simulink model "scar22"  (R2021a)
settings: Solver=ode23tb  StartTime=0.0  StopTime=.2  RelTol=1e-3
libraries: spsThreePhaseSeriesRLCLoadLib x17, spsThreePhasePISectionLineLib x16, spsThreePhaseTransformerTwoWindingsLib x14, spsThreePhaseVIMeasurementLib x11, simulink x6, exampleMicrogridLibrary x6, spsThreePhaseParallelRLCBranchLib x5, spsThreePhaseDynamicLoadLib x5, spsGroundLib x4, spsAC1AExcitationSystemLib x2, spsDieselMotorModel x2, spsSynchronousMachinepuStandardLib x2
(part 2 of 2)

== system scar22/Variable Load ==
  Load : Inport
  Dynamic Load Control : Subsystem
  Simple Three-Phase Load : spsThreePhaseDynamicLoadLib/Three-Phase Dynamic Load  NominalVoltage=[Vn Fn]  ActiveReactivePowers=[200000 45883.1]  PositiveSequence=[0.999844 -0.0038635]  ExternalControl=on  NpNq=[1.3 2]  TimeConstants="[0  0  0  0]"  MinimumVoltage=0.7  Tfilter=1e-2  LoadFlowParameters=[4,0,0,0,0]
      settings: SourceProductBaseCode=PS
  Terminator : Terminator
  A : PMIOPort  Side=Right
  B : PMIOPort  Port=2  Side=Right
  C : PMIOPort  Port=3  Side=Right
  wires:
  Simple Three-Phase Load/1 -> Terminator/1
  Load/1 -> Dynamic Load Control/1(P0)
  Dynamic Load Control/1(PQ) -> Simple Three-Phase Load/1
  connections:
  Simple Three-Phase Load/LConn1 -- A/RConn1
  Simple Three-Phase Load/LConn3 -- C/RConn1
  Simple Three-Phase Load/LConn2 -- B/RConn1

== system scar22/Diesel Generator1/Generator Measures ==
  m : Inport
  Bus Selector : BusSelector  OutputSignals="dq0 components.Stator voltage  vq (pu),dq0 components.Stator voltage  vd (pu)"  OutputAsBus=on
  Bus Selector1 : BusSelector  OutputSignals="Mechanical.Rotor speed  wm  (pu),dq0 components.Field current  ifd (pu)"
  Fcn1 : Fcn  Expr=sqrt(u(1)^2 + u(2)^2)
  Ifd : Outport  VectorParamsAs1DForOutWhenUnconnected=off
  Vt : Outport  Port=2  VectorParamsAs1DForOutWhenUnconnected=off
  wm : Outport  Port=3  VectorParamsAs1DForOutWhenUnconnected=off
  wires:
  Bus Selector1/2 -> Ifd/1  "<Field current  ifd (pu)>"
  Bus Selector/1 -> Fcn1/1
  Fcn1/1 -> Vt/1
  m/1 -> Bus Selector/1, Bus Selector1/1
  Bus Selector1/1 -> wm/1  "<Rotor speed  wm  (pu)>"

== system scar22/Diesel Generator1/Selected Measurements ==
  m : Inport
  Bus Creator : BusCreator  Inputs=7
  Bus Selector : BusSelector  OutputSignals="Mechanical.Electrical power  Pe (pu),Mechanical.Rotor speed  wm  (pu),Output active power   Peo (pu),Output reactive power  Qeo (pu)"
  to W : Gain  Gain=Pn
  to W1 : Gain  Gain=Pn
  to W2 : Gain  Gain=Pn
  sm : Outport  VectorParamsAs1DForOutWhenUnconnected=off
  wires:
  m/1 -> Bus Selector/1
  Bus Selector/4 -> to W2/1, Bus Creator/5  "<Output reactive power  Qeo (pu)>"
  Bus Selector/1 -> Bus Creator/2, to W/1  "<Electrical power  Pe (pu)>"
  Bus Selector/3 -> to W1/1, Bus Creator/4  "<Output active power   Peo (pu)>"
  to W/1 -> Bus Creator/1  "Electrical Power (W)"
  Bus Creator/1 -> sm/1
  Bus Selector/2 -> Bus Creator/3  "<Rotor speed  wm  (pu)>"
  to W1/1 -> Bus Creator/6  "Active Power (W)"
  to W2/1 -> Bus Creator/7  "Reactive Power (W)"

== system scar22/Diesel Generator2/Generator Measures ==
  m : Inport
  Bus Selector : BusSelector  OutputSignals="dq0 components.Stator voltage  vq (pu),dq0 components.Stator voltage  vd (pu)"  OutputAsBus=on
  Bus Selector1 : BusSelector  OutputSignals="Mechanical.Rotor speed  wm  (pu),dq0 components.Field current  ifd (pu)"
  Fcn1 : Fcn  Expr=sqrt(u(1)^2 + u(2)^2)
  Ifd : Outport  VectorParamsAs1DForOutWhenUnconnected=off
  Vt : Outport  Port=2  VectorParamsAs1DForOutWhenUnconnected=off
  wm : Outport  Port=3  VectorParamsAs1DForOutWhenUnconnected=off
  wires:
  Bus Selector1/2 -> Ifd/1  "<Field current  ifd (pu)>"
  Bus Selector/1 -> Fcn1/1
  Fcn1/1 -> Vt/1
  m/1 -> Bus Selector/1, Bus Selector1/1
  Bus Selector1/1 -> wm/1  "<Rotor speed  wm  (pu)>"

== system scar22/Diesel Generator2/Selected Measurements ==
  m : Inport
  Bus Creator : BusCreator  Inputs=7
  Bus Selector : BusSelector  OutputSignals="Mechanical.Electrical power  Pe (pu),Mechanical.Rotor speed  wm  (pu),Output active power   Peo (pu),Output reactive power  Qeo (pu)"
  to W : Gain  Gain=Pn
  to W1 : Gain  Gain=Pn
  to W2 : Gain  Gain=Pn
  sm : Outport  VectorParamsAs1DForOutWhenUnconnected=off
  wires:
  m/1 -> Bus Selector/1
  Bus Selector/4 -> to W2/1, Bus Creator/5  "<Output reactive power  Qeo (pu)>"
  Bus Selector/1 -> Bus Creator/2, to W/1  "<Electrical power  Pe (pu)>"
  Bus Selector/3 -> to W1/1, Bus Creator/4  "<Output active power   Peo (pu)>"
  to W/1 -> Bus Creator/1  "Electrical Power (W)"
  Bus Creator/1 -> sm/1
  Bus Selector/2 -> Bus Creator/3  "<Rotor speed  wm  (pu)>"
  to W1/1 -> Bus Creator/6  "Active Power (W)"
  to W2/1 -> Bus Creator/7  "Reactive Power (W)"

== system scar22/Energy Storage/Charge Limits ==
  SOC (%) : Inport
  Pin : Inport  Port=2
  Qin : Inport  Port=3
  Overcharge Check : Subsystem
  Undercharge Check : Subsystem
  Pbatt : Outport  VectorParamsAs1DForOutWhenUnconnected=off
  Qbatt : Outport  Port=2  VectorParamsAs1DForOutWhenUnconnected=off
  wires:
  SOC (%)/1 -> Overcharge Check/1(SOC (%)), Undercharge Check/1(SOC (%))
  Undercharge Check/2(Qout) -> Qbatt/1
  Pin/1 -> Overcharge Check/2(Pin)
  Overcharge Check/1(Pout) -> Undercharge Check/2(Pin)
  Qin/1 -> Overcharge Check/3(Qin)
  Undercharge Check/1(Pout) -> Pbatt/1  "Pbatt"
  Overcharge Check/2(Qout) -> Undercharge Check/3(Qin)

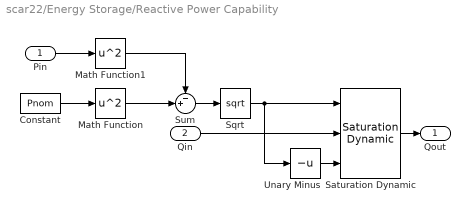
== system scar22/Energy Storage/Reactive Power Capability ==
  Pin : Inport
  Qin : Inport  Port=2
  Constant : Constant  Value=Pnom
  Math Function : Math  Operator=square  SignedPower=on  SaturateOnIntegerOverflow=on
  Math Function1 : Math  Operator=square  SignedPower=on  SaturateOnIntegerOverflow=on
  Saturation Dynamic : simulink/Discontinuities/Saturation Dynamic  OutMin=[]  OutMax=[]  OutDataTypeStr=Inherit: Same as second input  OutDataType=fixdt(1, 16)  OutScaling=2^-10  DoSatur=off
  Sqrt : Sqrt  SaturateOnIntegerOverflow=on
  Sum : Sum  Inputs=-+|
  Unary Minus : UnaryMinus
  Qout : Outport  VectorParamsAs1DForOutWhenUnconnected=off
  wires:
  Sqrt/1 -> Saturation Dynamic/1, Unary Minus/1
  Math Function1/1 -> Sum/1
  Math Function/1 -> Sum/2
  Constant/1 -> Math Function/1
  Sum/1 -> Sqrt/1
  Unary Minus/1 -> Saturation Dynamic/3
  Saturation Dynamic/1 -> Qout/1
  Pin/1 -> Math Function1/1
  Qin/1 -> Saturation Dynamic/2

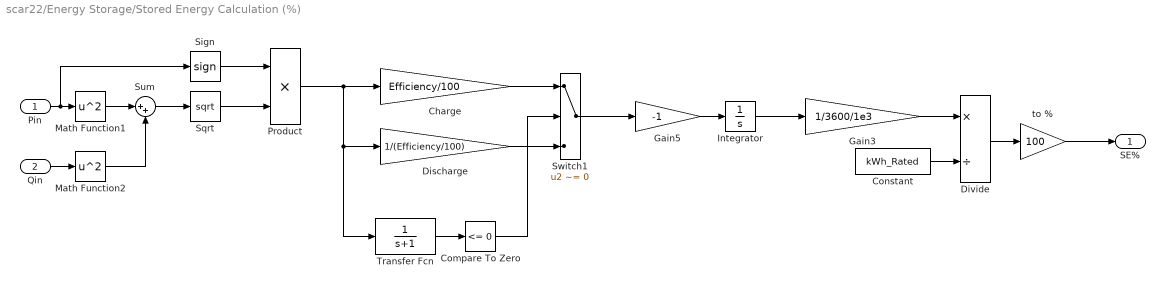
== system scar22/Energy Storage/Stored Energy Calculation (%) ==
  Pin : Inport
  Qin : Inport  Port=2
  Charge : Gain  Gain=Efficiency/100
  Compare To Zero : simulink/Logic and Bit Operations/Compare To Zero  relop=<=  OutDataTypeStr=boolean
  Constant : Constant  Value=kWh_Rated
  Discharge : Gain  Gain=1/(Efficiency/100)
  Divide : Product  Inputs=*/
  Gain3 : Gain  Gain=1/3600/1e3
  Gain5 : Gain  Gain=-1
  Integrator : Integrator  InitialCondition=(Initial_kWh_pc/100)*kWh_Rated*3600*1e3
  Math Function1 : Math  Operator=square  SignedPower=on  SaturateOnIntegerOverflow=on
  Math Function2 : Math  Operator=square  SignedPower=on  SaturateOnIntegerOverflow=on
  Product : Product
  Sign : Signum
  Sqrt : Sqrt  SaturateOnIntegerOverflow=on
  Sum : Sum  Inputs=|++
  Switch1 : Switch  Criteria=u2 ~= 0
  Transfer Fcn : TransferFcn  Denominator=[1 1]
  to % : Gain  Gain=100
  SE% : Outport  VectorParamsAs1DForOutWhenUnconnected=off
  wires:
  Sign/1 -> Product/1
  Sqrt/1 -> Product/2
  Sum/1 -> Sqrt/1
  Math Function2/1 -> Sum/2
  Math Function1/1 -> Sum/1
  Qin/1 -> Math Function2/1
  Pin/1 -> Math Function1/1, Sign/1
  Product/1 -> Transfer Fcn/1, Discharge/1, Charge/1
  Discharge/1 -> Switch1/3
  Gain5/1 -> Integrator/1
  to %/1 -> SE%/1
  Transfer Fcn/1 -> Compare To Zero/1
  Switch1/1 -> Gain5/1
  Gain3/1 -> Divide/1
  Constant/1 -> Divide/2
  Charge/1 -> Switch1/1
  Divide/1 -> to %/1
  Compare To Zero/1 -> Switch1/2
  Integrator/1 -> Gain3/1

== system scar22/Variable Load/Dynamic Load Control ==
  P0 : Inport
  Fcn : Fcn  Expr=sqrt(1/u(1)-1)
  Mux : Mux  Inputs=2
  Product : Product
  Summer1 : Constant  Value=PF
  PQ : Outport  VectorParamsAs1DForOutWhenUnconnected=off
  wires:
  Summer1/1 -> Fcn/1
  Fcn/1 -> Product/2
  P0/1 -> Product/1, Mux/1
  Mux/1 -> PQ/1
  Product/1 -> Mux/2  "Qo"

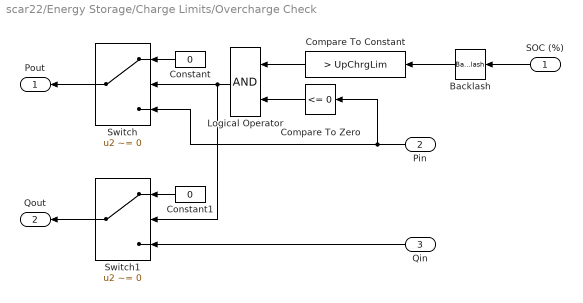
== system scar22/Energy Storage/Charge Limits/Overcharge Check ==
  SOC (%) : Inport
  Pin : Inport  Port=2
  Qin : Inport  Port=3
  Backlash : Backlash  BacklashWidth=1e-3  InitialOutput=Initial_kWh_pc  ZeroCross=off
  Compare To Constant : simulink/Logic and Bit Operations/Compare To Constant  relop=>  const=UpChrgLim  OutDataTypeStr=boolean
  Compare To Zero : simulink/Logic and Bit Operations/Compare To Zero  relop=<=  OutDataTypeStr=boolean
  Constant : Constant  Value=0
  Constant1 : Constant  Value=0
  Logical Operator : Logic  AllPortsSameDT=off  OutDataTypeStr=boolean
  Switch : Switch  Criteria=u2 ~= 0
  Switch1 : Switch  Criteria=u2 ~= 0
  Pout : Outport  VectorParamsAs1DForOutWhenUnconnected=off
  Qout : Outport  Port=2  VectorParamsAs1DForOutWhenUnconnected=off
  wires:
  Backlash/1 -> Compare To Constant/1
  Switch1/1 -> Qout/1
  Constant1/1 -> Switch1/1
  Qin/1 -> Switch1/3
  Compare To Zero/1 -> Logical Operator/2
  Switch/1 -> Pout/1
  Pin/1 -> Switch/3, Compare To Zero/1
  SOC (%)/1 -> Backlash/1
  Constant/1 -> Switch/1
  Logical Operator/1 -> Switch/2, Switch1/2
  Compare To Constant/1 -> Logical Operator/1

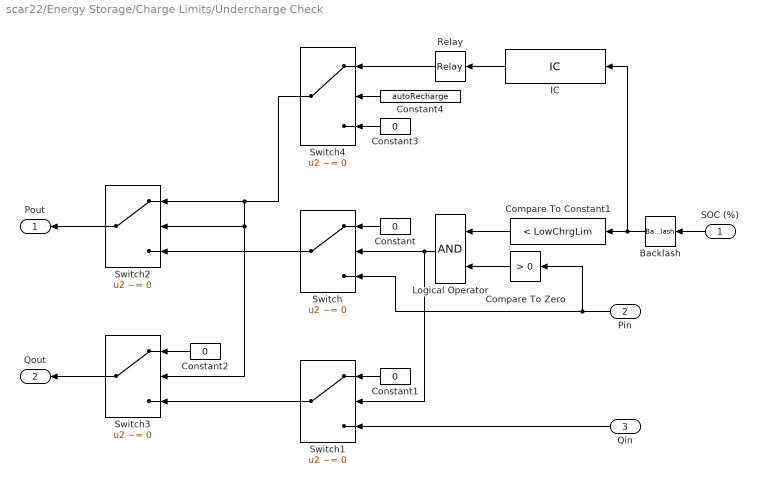
== system scar22/Energy Storage/Charge Limits/Undercharge Check ==
  SOC (%) : Inport
  Pin : Inport  Port=2
  Qin : Inport  Port=3
  Backlash : Backlash  BacklashWidth=1e-3  InitialOutput=Initial_kWh_pc  ZeroCross=off
  Compare To Constant1 : simulink/Logic and Bit Operations/Compare To Constant  relop=<  const=LowChrgLim  OutDataTypeStr=boolean
  Compare To Zero : simulink/Logic and Bit Operations/Compare To Zero  relop=>  OutDataTypeStr=boolean
  Constant{,1..3} (4 alike) : Constant  Value=0
  Constant4 : Constant  Value=autoRecharge
  IC : InitialCondition  Value=RechargeSOC
  Logical Operator : Logic  AllPortsSameDT=off  OutDataTypeStr=boolean
  Relay : Relay  OnSwitchValue=RechargeSOC  OffSwitchValue=LowChrgLim  OnOutputValue=0  OffOutputValue=-Precharge/100*Pnom
  Switch{,1..4} (5 alike) : Switch  Criteria=u2 ~= 0
  Pout : Outport  VectorParamsAs1DForOutWhenUnconnected=off
  Qout : Outport  Port=2  VectorParamsAs1DForOutWhenUnconnected=off
  wires:
  Constant4/1 -> Switch4/2
  Constant3/1 -> Switch4/3
  Relay/1 -> Switch4/1
  Constant2/1 -> Switch3/1
  Switch1/1 -> Switch3/3
  Switch3/1 -> Qout/1
  Switch2/1 -> Pout/1
  Switch/1 -> Switch2/3
  IC/1 -> Relay/1
  Switch4/1 -> Switch3/2, Switch2/2, Switch2/1
  Backlash/1 -> Compare To Constant1/1, IC/1
  Qin/1 -> Switch1/3
  Constant1/1 -> Switch1/1
  Compare To Constant1/1 -> Logical Operator/1
  Logical Operator/1 -> Switch1/2, Switch/2
  Constant/1 -> Switch/1
  SOC (%)/1 -> Backlash/1
  Pin/1 -> Compare To Zero/1, Switch/3
  Compare To Zero/1 -> Logical Operator/2
